simulink model "ClosedLoopStimPlexon"  (R2016b)
settings: Solver=FixedStepDiscrete  StartTime=0.0  StopTime=inf  FixedStep=sCoreParams.core.stepPeriod  RelTol=1e-3  EnableMultiTasking=on
values from neighbouring files (symbols this model uses):
  sCoreParams = InitCoreParams_Dependent(sCoreParams)    [initializationScript.m]
undefined symbols (not defined in the file or in its folder): daq
libraries: slrtlib x5, dspswit3 x3, daqlib x2, xpcnilib x2, simulink x1
settings Model: DataTypeOverride=Double  MinMaxOverflowLogging=ForceOff  Creator=rzelmann  LastModifiedBy=rzelmann
settings SolverCC: EnableConcurrentExecution=on  ConcurrentTasks=on
settings DataIOCC: SaveFormat=StructureWithTime
settings OptimizationCC: DefaultParameterBehavior=Inlined  EfficientFloat2IntCast=on  LifeSpan=inf
settings DebuggingCC: UniqueDataStoreMsg=error  StrictBusMsg=ErrorOnBusTreatedAsVector  SFUnexpectedBacktrackingDiag=warning  SFNoUnconditionalDefaultTransitionDiag=warning  SFExecutionAtInitializationDiag=none
settings HardwareCC: ProdBitPerPointer=32  ProdBitPerSizeT=32  ProdBitPerPtrDiffT=32  ProdLargestAtomicFloat=None  ProdWordSize=32  ProdLongLongMode=on  ProdHWDeviceType=Generic->32-bit x86 compatible
settings ModelReferenceCC: ModelReferenceNumInstancesAllowed=Single
settings RTWCC: SystemTargetFile=slrt.tlc  TLCOptions="-axPCMaxOverloads=30            -axPCOverLoadLen=2 -axPCStartupFlag=5"  TemplateMakefile=slrt_default_tmf  Description=Simulink Real-Time  RTWCompilerOptimization=on
settings CodeAppCC: MaxIdLength=63
settings ConfigComp: CovMetricSettings=dw  CovHtmlReporting=on  CovSaveCumulativeToWorkspaceVar=on  CovSaveSingleToWorkspaceVar=on  CovExternalEMLEnable=off

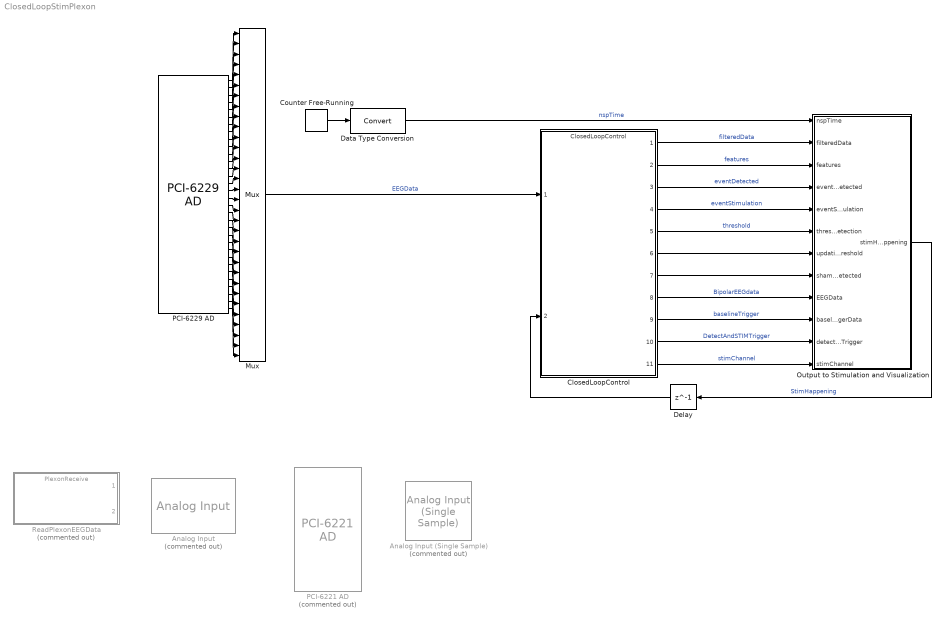
== system ClosedLoopStimPlexon ==
  Analog Input : daqlib/Analog Input  Commented=on  DeviceMenu=(none)  Device=ni Dev1 (USB-6009)  ObjConstructor=daq.createSession('ni')  NChannelsSelected=4  Channels=1$ai0$$Dev1$1$6$2$1$#1$ai1$$Dev1$1$6$2$1$#1$ai2$$Dev1$1$6$2$1$#1$ai3$$Dev1$1$6$2$1$#0$ai4$$Dev1$1$6$1$1$#0$ai5$$Dev1$1$6$1$1$#0$ai6$$Dev1$1$6$1$1$#0$ai7$$Dev1$1$6$1$1$#  NPorts=1 for all channels  SampleRate=2000  ActualRate=2000  ScansPerTrigger=100  OutputTimestamp=on  AcqMode=0  NumFrameBuffer=100  OutputTriggertime=off
  Analog Input (Single Sample) : daqlib/Analog Input (Single Sample)  Commented=on  DeviceMenu=(none)  Device=ni Dev1 (USB-6009)  ObjConstructor=daq.createSession('ni')  BlockSampleTime=.001  NChannelsSelected=8  Channels=1$ai0$$Dev1$1$6$1$1$#1$ai1$$Dev1$1$6$1$1$#1$ai2$$Dev1$1$6$1$1$#1$ai3$$Dev1$1$6$1$1$#1$ai4$$Dev1$1$7$1$1$#1$ai5$$Dev1$1$7$1$1$#1$ai6$$Dev1$1$7$1$1$#1$ai7$$Dev1$1$6$1$1$#  NPorts=1 for all channels  OutputTimestamp=on
  ClosedLoopControl : ModelReference  ModelNameDialog=ClosedLoopControl  SimulationMode=Normal  ModelReferenceVersion=1.661
  Counter Free-Running : simulink/Sources/Counter Free-Running  NumBits=64  tsamp=sCoreParams.core.stepPeriod
  Data Type Conversion : DataTypeConversion
  Delay : Delay  DelayLength=1  InitialCondition=0  InputProcessing=Columns as channels (frame based)  SampleTime=sCoreParams.core.stepPeriod
  Mux : Mux  Inputs=32
  Output to Stimulation and Visualization : Subsystem
  PCI-6221 AD : xpcnilib/A//D/M Series/PCI-6221 AD  Commented=on  channel=[1:16]  range=[5]  coupling=[0]  scantime=5e-6  sampletime=sCoreParams.core.stepPeriod  slot=-1
  PCI-6229 AD : xpcnilib/A//D/M Series/PCI-6229 AD  channel=[1:32]  range=[5]  coupling=[0]  scantime=5e-6  sampletime=sCoreParams.core.stepPeriod  slot=-1
  ReadPlexonEEGData : ModelReference  Commented=on  ModelNameDialog=PlexonReceive.slx  SimulationMode=Normal  ModelReferenceVersion=1.11
  wires:
  Output to Stimulation and Visualization/1(stimHappening) -> Delay/1  "StimHappening"
  Mux/1 -> ClosedLoopControl/1  "EEGData"
  ClosedLoopControl/1 -> Output to Stimulation and Visualization/2(filteredData)  "filteredData"
  Data Type Conversion/1 -> Output to Stimulation and Visualization/1(nspTime)  "nspTime"
  ClosedLoopControl/4 -> Output to Stimulation and Visualization/5(eventStimulation)  "eventStimulation"
  ClosedLoopControl/6 -> Output to Stimulation and Visualization/7(updatingThreshold)
  ClosedLoopControl/8 -> Output to Stimulation and Visualization/9(EEGData)  "BipolarEEGdata"
  ClosedLoopControl/9 -> Output to Stimulation and Visualization/10(baselineTriggerData)  "baselineTrigger"
  ClosedLoopControl/10 -> Output to Stimulation and Visualization/11(detectStimTrigger)  "DetectAndSTIMTrigger"
  Delay/1 -> ClosedLoopControl/2
  ClosedLoopControl/11 -> Output to Stimulation and Visualization/12(stimChannel)  "stimChannel"
  ClosedLoopControl/7 -> Output to Stimulation and Visualization/8(shamDetected)
  ClosedLoopControl/5 -> Output to Stimulation and Visualization/6(thresholdUsedInDetection)  "threshold"
  ClosedLoopControl/3 -> Output to Stimulation and Visualization/4(eventDetected)  "eventDetected"
  ClosedLoopControl/2 -> Output to Stimulation and Visualization/3(features)  "features"
  PCI-6229 AD/1 -> Mux/1
  PCI-6229 AD/2 -> Mux/2
  PCI-6229 AD/3 -> Mux/3
  PCI-6229 AD/4 -> Mux/4
  PCI-6229 AD/5 -> Mux/5
  PCI-6229 AD/6 -> Mux/6
  PCI-6229 AD/7 -> Mux/7
  PCI-6229 AD/8 -> Mux/8
  PCI-6229 AD/9 -> Mux/9
  PCI-6229 AD/10 -> Mux/10
  PCI-6229 AD/11 -> Mux/11
  PCI-6229 AD/12 -> Mux/12
  PCI-6229 AD/13 -> Mux/13
  PCI-6229 AD/14 -> Mux/14
  PCI-6229 AD/15 -> Mux/15
  PCI-6229 AD/16 -> Mux/16
  PCI-6229 AD/17 -> Mux/17
  PCI-6229 AD/18 -> Mux/18
  PCI-6229 AD/19 -> Mux/19
  PCI-6229 AD/20 -> Mux/20
  PCI-6229 AD/21 -> Mux/21
  PCI-6229 AD/22 -> Mux/22
  PCI-6229 AD/23 -> Mux/23
  PCI-6229 AD/24 -> Mux/24
  PCI-6229 AD/25 -> Mux/25
  PCI-6229 AD/26 -> Mux/26
  PCI-6229 AD/27 -> Mux/27
  PCI-6229 AD/28 -> Mux/28
  PCI-6229 AD/29 -> Mux/29
  PCI-6229 AD/30 -> Mux/30
  PCI-6229 AD/31 -> Mux/31
  PCI-6229 AD/32 -> Mux/32
  Counter Free-Running/1 -> Data Type Conversion/1

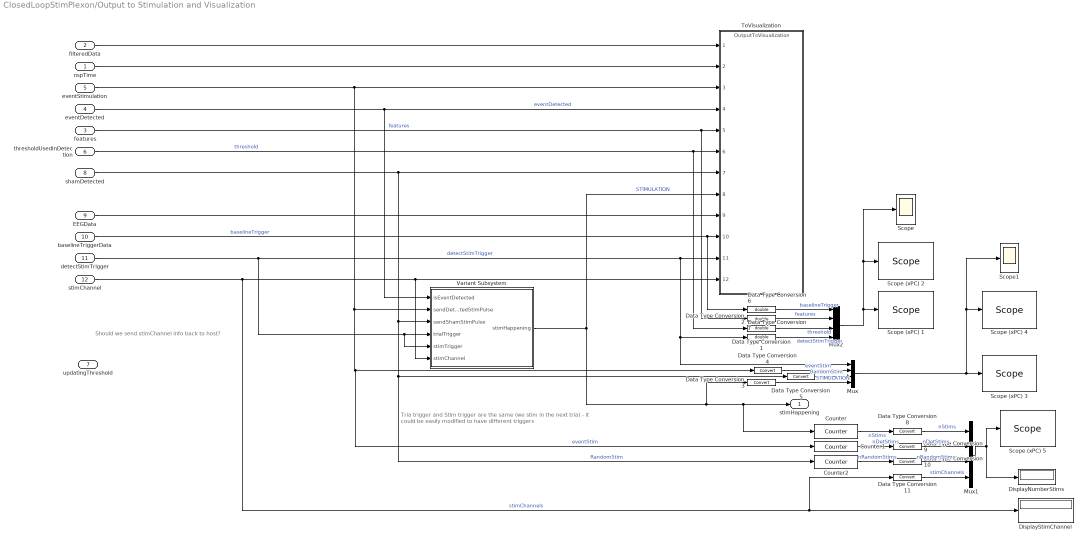
== system ClosedLoopStimPlexon/Output to Stimulation and Visualization ==
  note: Should we send stimChannel info back to host?
  note: Tria trigger and Stim trigger are the same (we stim in the next tria)
      | - it could be easily modified to have different triggers
  nspTime : Inport
  filteredData : Inport  Port=2
  features : Inport  Port=3
  eventDetected : Inport  Port=4
  eventStimulation : Inport  Port=5
  thresholdUsedInDetection : Inport  Port=6
  updatingThreshold : Inport  Port=7
  shamDetected : Inport  Port=8
  EEGData : Inport  Port=9
  baselineTriggerData : Inport  Port=10  OutDataTypeStr=int32
  detectStimTrigger : Inport  Port=11  OutDataTypeStr=int32
  stimChannel : Inport  Port=12
  Counter : dspswit3/Counter  Direction=Up  CountEvent=Rising edge  CounterSize=User defined  MaxCount=1024  InitialCount=0  Output=Count  HitValue=32  ResetInput=off  SamplesPerFrame=1  Ts=1  CntDtype=int32  HitDtype=Logical
  Counter1 : dspswit3/Counter  Direction=Up  CountEvent=Rising edge  CounterSize=User defined  MaxCount=1024  InitialCount=0  Output=Count  HitValue=32  ResetInput=off  SamplesPerFrame=1  Ts=1  CntDtype=int32  HitDtype=Logical
  Counter2 : dspswit3/Counter  Direction=Up  CountEvent=Rising edge  CounterSize=User defined  MaxCount=1024  InitialCount=0  Output=Count  HitValue=32  ResetInput=off  SamplesPerFrame=1  Ts=1  CntDtype=int32  HitDtype=Logical
  Data Type Conversion{1..2,6..7} (4 alike) : DataTypeConversion  OutDataTypeStr=double
  Data Type Conversion{3..5,8..11} (7 alike) : DataTypeConversion
  DisplayNumberStims : Display
  DisplayStimChannel : Display
  Mux : Mux
  Mux1 : Mux
  Mux2 : Mux
  Scope : Scope
  Scope (xPC) 1 : slrtlib/Displays and Logging/Scope   scopeno=1  scopetype=Target  autostart=on  viewmode=Graphical sliding  formatstr='%15.6f'  grid=on  ylimits=[0,0]  nosamples=1000  noprepostsamples=0  interleave=1  triggermode=FreeRun  triggersignal=1  trigsignalfromport=on  triggerlevel=0.0  triggerslope=Rising  triggerscope=1  triggersample=0  filename=data.dat  mode=Lazy  writesize=512  autorestart=off  dynamicfilemode=off  maxwritefilesize=512*1024^2
  Scope (xPC) 2 : slrtlib/Displays and Logging/Scope   scopeno=2  scopetype=File  autostart=on  viewmode=Graphical redraw  formatstr='%15.6f'  grid=on  ylimits=[0,0]  nosamples=1000  noprepostsamples=-10  interleave=1  triggermode=FreeRun  triggersignal=1  trigsignalfromport=on  triggerlevel=0.0  triggerslope=Rising  triggerscope=1  triggersample=0  filename=featTh.dat  mode=Lazy  writesize=512  autorestart=off  dynamicfilemode=off  maxwritefilesize=512*1024^2
  Scope (xPC) 3 : slrtlib/Displays and Logging/Scope   scopeno=3  scopetype=Target  autostart=on  viewmode=Graphical sliding  formatstr='%15.6f'  grid=on  ylimits=[0,0]  nosamples=1000  noprepostsamples=0  interleave=1  triggermode=FreeRun  triggersignal=1  trigsignalfromport=on  triggerlevel=0.0  triggerslope=Rising  triggerscope=1  triggersample=0  filename=data.dat  mode=Lazy  writesize=512  autorestart=off  dynamicfilemode=off  maxwritefilesize=512*1024^2
  Scope (xPC) 4 : slrtlib/Displays and Logging/Scope   scopeno=4  scopetype=File  autostart=on  viewmode=Graphical redraw  formatstr='%15.6f'  grid=on  ylimits=[0,0]  nosamples=1000  noprepostsamples=-10  interleave=1  triggermode=FreeRun  triggersignal=1  trigsignalfromport=on  triggerlevel=0.0  triggerslope=Rising  triggerscope=1  triggersample=0  filename=detStim.dat  mode=Lazy  writesize=512  autorestart=off  dynamicfilemode=off  maxwritefilesize=512*1024^2
  Scope (xPC) 5 : slrtlib/Displays and Logging/Scope   scopeno=5  scopetype=Target  autostart=on  viewmode=Numerical  formatstr='%d'  grid=on  ylimits=[0,0]  nosamples=1000  noprepostsamples=0  interleave=1  triggermode=FreeRun  triggersignal=1  trigsignalfromport=on  triggerlevel=0.0  triggerslope=Rising  triggerscope=1  triggersample=0  filename=data.dat  mode=Lazy  writesize=512  autorestart=off  dynamicfilemode=off  maxwritefilesize=512*1024^2
  Scope1 : Scope
  ToVisualization : ModelReference  ModelNameDialog=OutputToVisualization  SimulationMode=Normal  ModelReferenceVersion=1.235
  Variant Subsystem : Subsystem  Variant=on
  stimHappening : Outport  OutDataTypeStr=boolean  SampleTime=sCoreParams.core.stepPeriod
  wires:
  eventDetected/1 -> Variant Subsystem/1(isEventDetected), ToVisualization/4  "eventDetected"
  nspTime/1 -> ToVisualization/2
  shamDetected/1 -> Counter2/1, Data Type Conversion5/1, Variant Subsystem/3(sendShamStimPulse), ToVisualization/7  "RandomStim"
  Variant Subsystem/1(stimHappening) -> ToVisualization/8, Data Type Conversion3/1, Counter/1, stimHappening/1  "STIMULATION"
  eventStimulation/1 -> ToVisualization/3, Variant Subsystem/2(sendDetectedStimPulse), Data Type Conversion4/1, Counter1/1  "eventStim"
  filteredData/1 -> ToVisualization/1
  EEGData/1 -> ToVisualization/9
  features/1 -> Data Type Conversion2/1, ToVisualization/5  "features"
  thresholdUsedInDetection/1 -> Data Type Conversion1/1, ToVisualization/6  "threshold"
  Data Type Conversion3/1 -> Mux/4  "STIMULATION"
  Data Type Conversion4/1 -> Mux/2  "eventStim"
  Mux2/1 -> Scope/1, Scope (xPC) 2/1, Scope (xPC) 1/1
  Mux/1 -> Scope1/1, Scope (xPC) 4/1, Scope (xPC) 3/1
  Data Type Conversion5/1 -> Mux/3  "RandomStim"
  baselineTriggerData/1 -> Data Type Conversion6/1, ToVisualization/10  "baselineTrigger"
  Data Type Conversion1/1 -> Mux2/3  "threshold"
  Data Type Conversion2/1 -> Mux2/2  "features"
  Data Type Conversion6/1 -> Mux2/1  "baselineTrigger"
  detectStimTrigger/1 -> Variant Subsystem/5(stimTrigger), Variant Subsystem/4(trialTrigger), Mux/1, Data Type Conversion7/1, ToVisualization/11  "detectStimTrigger"
  Data Type Conversion7/1 -> Mux2/4  "detectStimTrigger"
  stimChannel/1 -> Variant Subsystem/6(stimChannel), ToVisualization/12, Data Type Conversion11/1, DisplayStimChannel/1  "stimChannels"
  Counter/1 -> Data Type Conversion8/1  "nStims"
  Mux1/1 -> Scope (xPC) 5/1, DisplayNumberStims/1
  Counter1/1 -> Data Type Conversion9/1  "nDetStims"
  Counter2/1 -> Data Type Conversion10/1  "nRandomStims"
  Data Type Conversion8/1 -> Mux1/1  "nStims"
  Data Type Conversion9/1 -> Mux1/2  "nDetStims"
  Data Type Conversion10/1 -> Mux1/3  "nRandomStims"
  Data Type Conversion11/1 -> Mux1/4  "stimChannels"

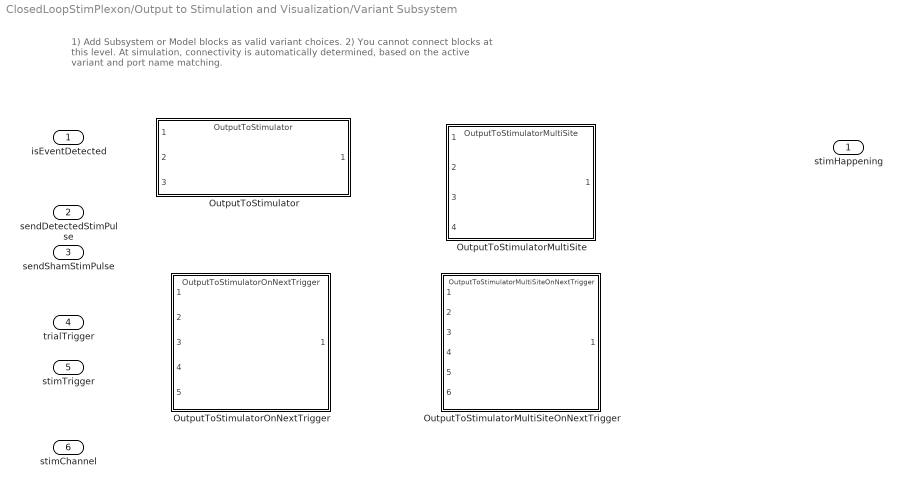
== system ClosedLoopStimPlexon/Output to Stimulation and Visualization/Variant Subsystem ==
  note: 1) Add Subsystem or Model blocks as valid variant choices.
      | 2) You cannot connect blocks at this level. At simulation, connectivity is automatically
      | determined, based on the active variant and port name matching.
  isEventDetected : Inport
  sendDetectedStimPulse : Inport  Port=2
  sendShamStimPulse : Inport  Port=3
  trialTrigger : Inport  Port=4
  stimTrigger : Inport  Port=5
  stimChannel : Inport  Port=6  OutDataTypeStr=int32
  OutputToStimulator : ModelReference  ModelNameDialog=OutputToStimulator  SimulationMode=Normal  VariantControl=variantParams_STIMULATION_REALTIME  ModelReferenceVersion=1.30
  OutputToStimulatorMultiSite : ModelReference  ModelNameDialog=OutputToStimulatorMultiSite.slx  SimulationMode=Normal  VariantControl=variantParams_STIMULATION_MULTISITE_REALTIME  ModelReferenceVersion=1.45
  OutputToStimulatorMultiSiteOnNextTrigger : ModelReference  ModelNameDialog=OutputToStimulatorMultiSiteOnNextTrigger.slx  SimulationMode=Normal  VariantControl=variantParams_STIMULATION_MULTISITE_NEXTTRIGGER  ModelReferenceVersion=1.63
  OutputToStimulatorOnNextTrigger : ModelReference  ModelNameDialog=OutputToStimulatorOnNextTrigger  SimulationMode=Normal  VariantControl=variantParams_STIMULATION_ONNEXTTRIGGER  ModelReferenceVersion=1.45
  stimHappening : Outport
